simulink model "COBEM_SIMULINK_OFICIAL"  (R2018a)
settings: Solver=ode4  StartTime=0.0  StopTime=tfinal  FixedStep=dt  RelTol=1e-3
values from neighbouring files (symbols this model uses):
  a1 = num1/den1    (= 0.0190125110732)    [COBEM_Oficial.m]
  a2 = num2/den2    [COBEM_Oficial.m]
  a3 = num3/den3    [COBEM_Oficial.m]
  a4 = num4/den4    [COBEM_Oficial.m]
  h10 = 0.25    [COBEM_Oficial.m]
  H1max = 1    [COBEM_Oficial.m]
  h20 = 0.25    [COBEM_Oficial.m]
  h2_G = (ones(2501           ,1))*0.75    [COBEM_Oficial.m]
  H2max = 1    [COBEM_Oficial.m]
  Kd = sol(3)    [COBEM_Oficial.m]
  Ki = sol(2)    [COBEM_Oficial.m]
  Kp = sol(1)    [COBEM_Oficial.m]
  N = 100    [COBEM_Oficial.m]
settings Model: Creator=generic-user  LastModifiedBy=generic-user

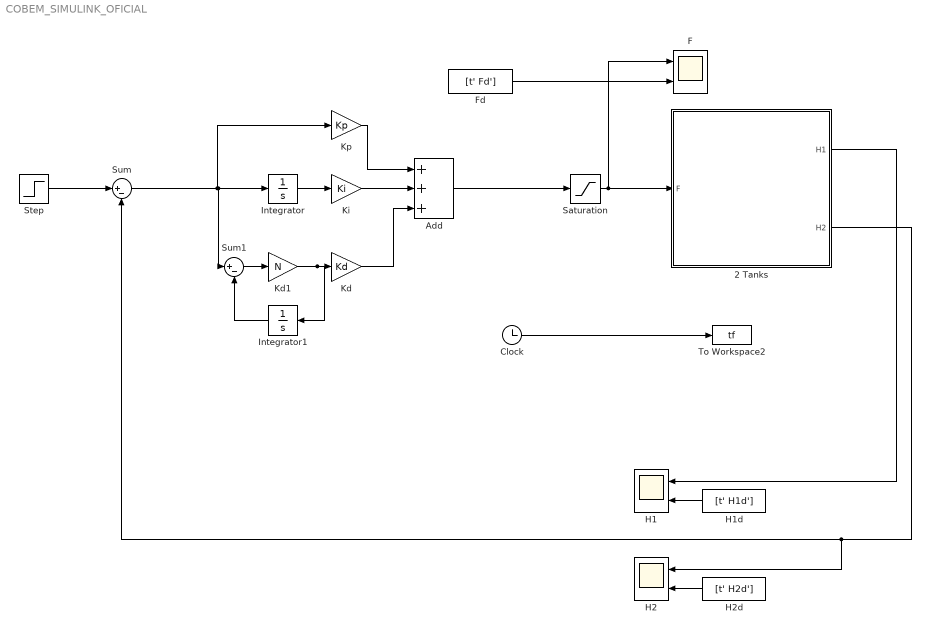
== system COBEM_SIMULINK_OFICIAL ==
  2 Tanks : Subsystem
  Add : Sum  Inputs=+++
  Clock : Clock
  F : Scope  NumInputPorts=2
  Fd : FromWorkspace  VariableName=[t' Fd']  SampleTime=0  OutputAfterFinalValue=Holding final value
  H1 : Scope  NumInputPorts=2
  H1d : FromWorkspace  VariableName=[t' H1d']  SampleTime=0  OutputAfterFinalValue=Holding final value
  H2 : Scope  NumInputPorts=2
  H2d : FromWorkspace  VariableName=[t' H2d']  SampleTime=0  OutputAfterFinalValue=Holding final value
  Integrator : Integrator
  Integrator1 : Integrator
  Kd : Gain  Gain=Kd
  Kd1 : Gain  Gain=N
  Ki : Gain  Gain=Ki
  Kp : Gain  Gain=Kp
  Saturation : Saturate  UpperLimit=90  LowerLimit=0
  Step : Step  Time=0  After=h2_G(1)  SampleTime=0
  Sum : Sum  Inputs=|+-
  Sum1 : Sum  Inputs=|+-
  To Workspace2 : ToWorkspace  VariableName=tf  SampleTime=-1
  wires:
  H1d/1 -> H1/2
  Clock/1 -> To Workspace2/1
  H2d/1 -> H2/2
  2 Tanks/1(H1) -> H1/1
  2 Tanks/2(H2) -> Sum/2, H2/1
  Fd/1 -> F/2
  Integrator/1 -> Ki/1
  Add/1 -> Saturation/1
  Saturation/1 -> F/1, 2 Tanks/1(F)
  Kd/1 -> Add/3
  Ki/1 -> Add/2
  Kp/1 -> Add/1
  Step/1 -> Sum/1
  Sum/1 -> Kp/1, Sum1/1, Integrator/1
  Integrator1/1 -> Sum1/2
  Sum1/1 -> Kd1/1
  Kd1/1 -> Integrator1/1, Kd/1

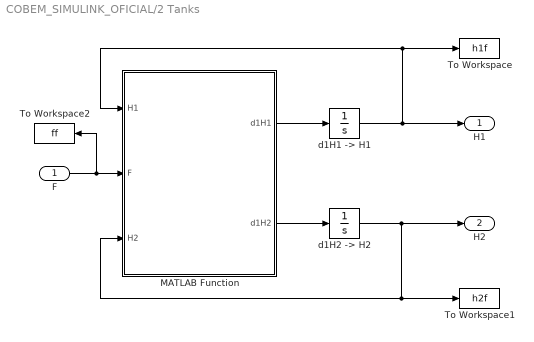
== system COBEM_SIMULINK_OFICIAL/2 Tanks ==
  F : Inport
  MATLAB Function : MATLAB Function  TreatAsAtomicUnit=on
  To Workspace : ToWorkspace  VariableName=h1f  SampleTime=-1
  To Workspace1 : ToWorkspace  VariableName=h2f  SampleTime=-1
  To Workspace2 : ToWorkspace  VariableName=ff  SampleTime=-1
  "d1H1 -> H1" : Integrator  InitialCondition=h10  LimitOutput=on  UpperSaturationLimit=H1max  LowerSaturationLimit=0
  "d1H2 -> H2" : Integrator  InitialCondition=h20  LimitOutput=on  UpperSaturationLimit=H2max  LowerSaturationLimit=0
  H1 : Outport
  H2 : Outport  Port=2
  wires:
  MATLAB Function/1(d1H1) -> "d1H1 -> H1"/1
  "d1H1 -> H1"/1 -> H1/1, To Workspace/1, MATLAB Function/1(H1)
  MATLAB Function/2(d1H2) -> "d1H2 -> H2"/1
  F/1 -> To Workspace2/1, MATLAB Function/2(F)
  "d1H2 -> H2"/1 -> H2/1, To Workspace1/1, MATLAB Function/3(H2)

== matlab function COBEM_SIMULINK_OFICIAL/2 Tanks/MATLAB Function ==
  data: H1 input; F input; d1H1 output; H2 input; d1H2 output; a1 parameter; a2 parameter; a3 parameter; a4 parameter
function [d1H1, d1H2] = TwoTanks(H1, F, H2, a1, a2, a3, a4)
  
  % Sistema Dinâmico
    d1H1 = a1*F - a2*sqrt(H1);
    
    d1H2 = a3*(sqrt(H1)/(H2^2)) - a4*(1/(H2^1.5));
